simulink model "ImageTest"  (R2015b)
settings: Solver=VariableStepAuto  StartTime=0.0  StopTime=inf  RelTol=1e-3
undefined symbols (not defined in the file): externalTrigger, fallingEdge, gray, IsPositionTracked, IsSkeletonTracked, JointDepthIndices, JointImageIndices, JointTrackingState, JointWorldCoordinates, PositionDepthIndices, PositionImageIndices, PositionWorldCoordinates, SegmentationData, SkeletonTrackingID, videoinput
libraries: visionconversions x1, visionstatistics x1, imaqlib x1, visionsinks x1, simulink x1
settings Model: Creator=henry  LastModifiedBy=henry

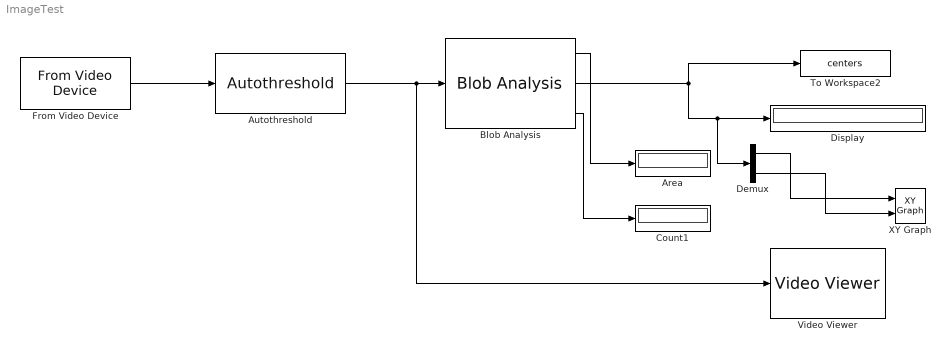
== system ImageTest ==
  Area : Display
  Autothreshold : visionconversions/Autothreshold  operator=>  threshOut=off  effMetricOut=off  userDefinedRange=off  umin=0  umax=255  outOfRngOpt=Warn and saturate  scaleThreshold=off  scaleFactor=1  P1Mode=Specify word length  P1WordLength=32  P1FracLength=30  P2Mode=Specify word length  P2WordLength=32  P2FracLength=22  P3Mode=Specify word length  P3WordLength=32  P3FracLength=14  P4Mode=Binary point scaling  P4WordLength=32  P4FracLength=15  Q1Mode=Specify word length  Q1WordLength=32  Q1FracLength=16  EMMode=Specify word length  EMWordLength=16  EMFracLength=14  roundingMode=Floor  overflowMode=off
  Blob Analysis : visionstatistics/Blob Analysis  Tag=vipblks_row_conv  area=on  centroid=on  bBox=off  majorAxis=off  minorAxis=off  angle=off  eccentricity=off  equivDiameterSq=off  extent=off  perimeter=off  maxBlobs=1  warnIfNumBlobsExceeded=off  isCount=on  useMinArea=off  minArea=200000  useMaxArea=off  maxArea=350000  excludeBorderBlob=on  outDT=double  isOutVarDim=off  isFill=off  fillValues=-1  conn=8  isLabel=off  outputMode=Binary point scaling  outputWordLength=32  outputFracLength=16  firstCoeffMode=Binary point scaling  firstCoeffWordLength=16  firstCoeffFracLength=14  secondCoeffMode=Binary point scaling  secondCoeffWordLength=32  secondCoeffFracLength=16  accumMode=Binary point scaling  accumWordLength=32  accumFracLength=0  prodOutputMode=Binary point scaling  prodOutputWordLength=32  prodOutputFracLength=16  roundingMode=Floor  overflowMode=off
  Count1 : Display
  Demux : Demux  Outputs=2
  Display : Display
  From Video Device : imaqlib/From Video Device  DeviceMenu=dcam 1 (FO134SB)  Device=dcam 1 (FO134SB)  ObjConstructor=videoinput('dcam', 1)  VideoFormatMenu=F7_Y8_640x480_mode0  VideoFormat=F7_Y8_640x480_mode0  VideoSource=default  ROIPosition=[0 0 480 640]  EnableHWTrigger=off  TriggerConfiguration=externalTrigger/fallingEdge  SampleTime=1/30  OutputPortsMode=One multidimensional signal  DataType=single  CanDoHWTrigger=yes  ReturnedColorSpace=grayscale  BlockHandle=2054.0007  ROIWidth=640  ROIHeight=480  ROIColumn=0  ROIRow=0  EngXMLPath=/home/henry/Matlab2015b/toolbox/imaq/imaq/private  DevXMLPath=/home/henry/Documents/MATLAB/SupportPackages/R2015b/dcamhardware/toolbox/imaq/supportpackages/dcam/adaptor/glnxa64  EngLibPath=/home/henry/Matlab2015b/toolbox/imaq/imaqblks/imaqmex/glnxa64  ColorSpace=grayscale  BayerSensorAlignment=grbg  AllMetadata=IsPositionTracked;IsSkeletonTracked;JointDepthIndices;JointImageIndices;JointTrackingState;JointWorldCoordinates;PositionDepthIndices;PositionImageIndices;PositionWorldCoordinates;SegmentationData;SkeletonTrackingID
  To Workspace2 : ToWorkspace  VariableName=centers  SampleTime=-1
  Video Viewer : visionsinks/Video Viewer  inputType=Obsolete7b  imagePorts=One multidimensional signal  useColorMap=off  colormapValue=gray(256)  specRange=off  minInputVal=0  maxInputVal=255  FigPos=[176 754 965 524]  AxisZoom=on  trueSizedOnce=off  OpenAtMdlStart=on  DefaultConfigurationName=vipscopes.VideoViewerScopeCfg
  XY Graph : simulink/Sinks/XY Graph  xmin=0  xmax=700  ymin=0  ymax=700  st=-1
  wires:
  Autothreshold/1 -> Video Viewer/1, Blob Analysis/1
  Demux/1 -> XY Graph/1
  Demux/2 -> XY Graph/2
  From Video Device/1 -> Autothreshold/1
  Blob Analysis/1 -> Area/1
  Blob Analysis/2 -> Demux/1, Display/1, To Workspace2/1
  Blob Analysis/3 -> Count1/1
